simulink model "invdyn_control_test"  (R2024b)
settings: Solver=ode1  StartTime=0.0  StopTime=50  FixedStep=dt  RelTol=1e-3
model workspace (MAT data in the model file):
  dt = 0.001
libraries: sdu_controllers x6, robotcorelib x2
settings Model: Creator=eld  LastModifiedBy=eld

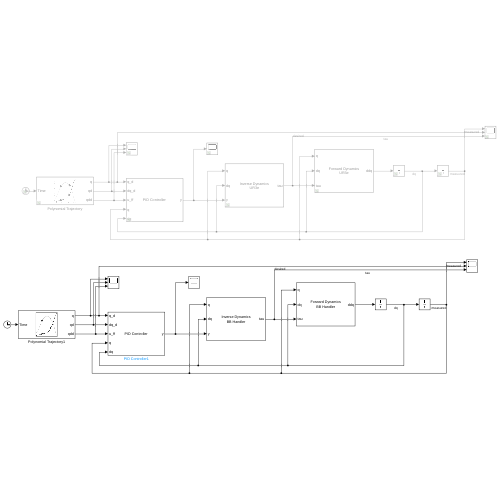
[thumbnail: Simulink's stored preview of the top-level diagram]
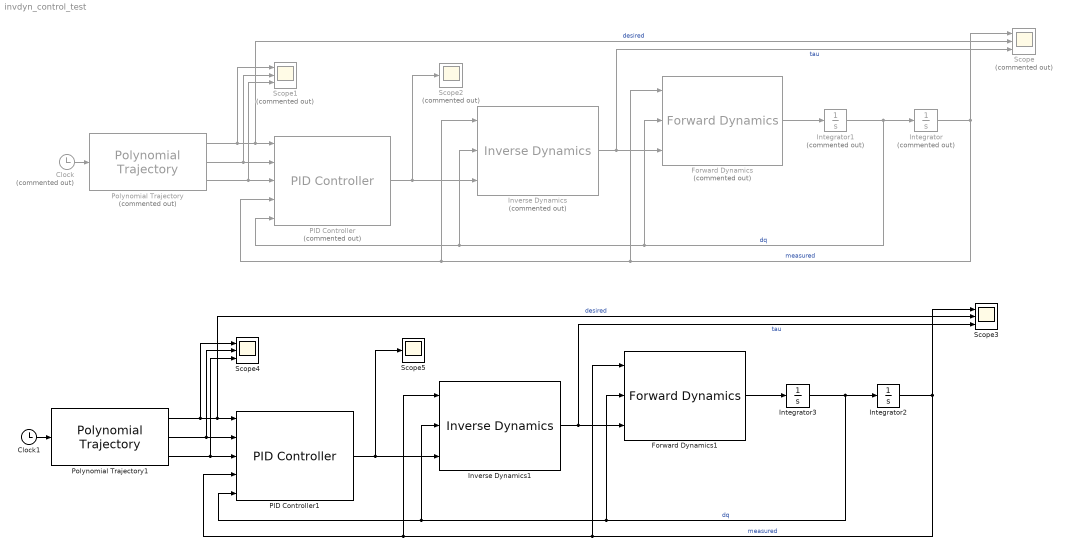
== system invdyn_control_test ==
  " Inverse Dynamics" : sdu_controllers/ Inverse Dynamics  Commented=on  RobotType=UR3e  SimulateUsing=Interpreted execution
  " Inverse Dynamics1" : sdu_controllers/ Inverse Dynamics  RobotType=BB Handler  SimulateUsing=Interpreted execution
  Clock : Clock  Commented=on
  Clock1 : Clock
  Forward Dynamics : sdu_controllers/Forward Dynamics  Commented=on  RobotType=UR3e  SimulateUsing=Interpreted execution
  Forward Dynamics1 : sdu_controllers/Forward Dynamics  RobotType=BB Handler  SimulateUsing=Interpreted execution
  Integrator : Integrator  Commented=on  InitialCondition=[0;-pi/2;-pi/2;-pi/2;pi/2;0]
  Integrator1 : Integrator  Commented=on  InitialCondition=zeros(6,1)
  Integrator2 : Integrator  InitialCondition=[0;-pi/2;-pi/2;-pi/2;pi/2;0; pi/2]
  Integrator3 : Integrator  InitialCondition=zeros(7,1)
  PID Controller : sdu_controllers/PID Controller  Commented=on  Kp=100.0  Ki=0  Kd=2*sqrt(100)  N=1  num_states=6  sample_time=dt  SimulateUsing=Interpreted execution
  PID Controller1 : sdu_controllers/PID Controller  Kp=100.0  Ki=0  Kd=2*sqrt(100)  N=1  num_states=7  sample_time=dt  SimulateUsing=Interpreted execution
  Polynomial Trajectory : robotcorelib/Polynomial Trajectory  Commented=on  WaypointSource=Internal  Waypoints="[0, -pi/2, -pi/2, -pi/2, pi/2, 0;  deg2rad(45), deg2rad(-120), -pi/2, deg2rad(-60), pi/2, deg2rad(-45); -1, pi/2, pi/2, pi/2, -pi/2, 1].'"  TimePoints=[ 0, 25, 50]  TimeInterval=[ 1, 4 ]  Method=Quintic Polynomial  ParameterSource=Internal  VelocityBoundaryCondition=zeros( 6, 3)  AccelerationBoundaryCondition=zeros( 6,3)  SimulateUsing=Code generation
  Polynomial Trajectory1 : robotcorelib/Polynomial Trajectory  WaypointSource=Internal  Waypoints="[0, -pi/2, -pi/2, -pi/2, pi/2, 0, pi/2;  deg2rad(45), deg2rad(-120), -pi/2, deg2rad(-60), pi/2, deg2rad(-45), 0; -1, pi/2, pi/2, pi/2, -pi/2, 1, -pi/2].'"  TimePoints=[ 0, 25, 50]  TimeInterval=[ 1, 4 ]  Method=Quintic Polynomial  ParameterSource=Internal  VelocityBoundaryCondition=zeros( 7, 3)  AccelerationBoundaryCondition=zeros( 7,3)  SimulateUsing=Code generation
  Scope : Scope  Commented=on  NumInputPorts=3
  Scope1 : Scope  Commented=on  NumInputPorts=3
  Scope2 : Scope  Commented=on
  Scope3 : Scope  NumInputPorts=3
  Scope4 : Scope  NumInputPorts=3
  Scope5 : Scope
  wires:
  Integrator1/1 -> Integrator/1, PID Controller/5, " Inverse Dynamics"/2, Forward Dynamics/2  "dq"
  Integrator/1 -> Scope/1, PID Controller/4, " Inverse Dynamics"/1, Forward Dynamics/1  "measured"
  PID Controller/1 -> Scope2/1, " Inverse Dynamics"/3
  " Inverse Dynamics"/1 -> Scope/3, Forward Dynamics/3  "tau"
  Polynomial Trajectory/1 -> Scope1/1, Scope/2, PID Controller/1  "desired"
  Polynomial Trajectory/2 -> Scope1/2, PID Controller/2
  Polynomial Trajectory/3 -> Scope1/3, PID Controller/3
  Clock/1 -> Polynomial Trajectory/1
  Forward Dynamics/1 -> Integrator1/1
  " Inverse Dynamics1"/1 -> Scope3/3, Forward Dynamics1/3  "tau"
  Polynomial Trajectory1/2 -> Scope4/2, PID Controller1/2
  PID Controller1/1 -> Scope5/1, " Inverse Dynamics1"/3
  Polynomial Trajectory1/3 -> Scope4/3, PID Controller1/3
  Polynomial Trajectory1/1 -> Scope4/1, Scope3/2, PID Controller1/1  "desired"
  Integrator2/1 -> Scope3/1, PID Controller1/4, " Inverse Dynamics1"/1, Forward Dynamics1/1  "measured"
  Integrator3/1 -> Integrator2/1, PID Controller1/5, " Inverse Dynamics1"/2, Forward Dynamics1/2  "dq"
  Forward Dynamics1/1 -> Integrator3/1
  Clock1/1 -> Polynomial Trajectory1/1
